simulink library "ESTS_TFY"  (R2023b)
settings: Solver=VariableStepAuto  StartTime=0.0  StopTime=10.0  RelTol=1e-3
libraries: ESTS_TFY_YawMomFromFx x1, ESTS_TFY_LatForceFromFx x1, ESTS_TFY_LatAxle x1, ESTS_TFY_FLatTir x1
settings Model: Creator=blatak  LastModifiedBy=blatak
settings ModelReferenceCC: EnableRefExpFcnMdlSchedulingChecks=on

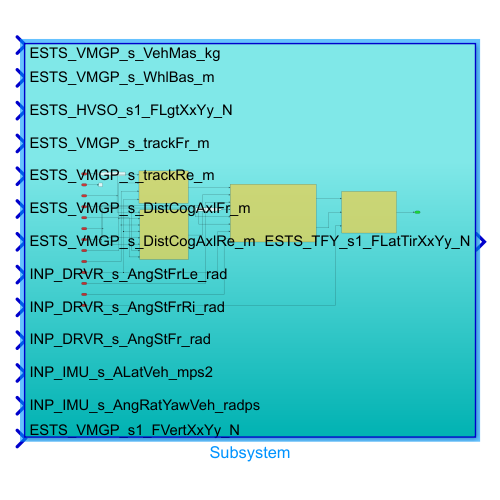
[thumbnail: Simulink's stored preview of the top-level diagram]
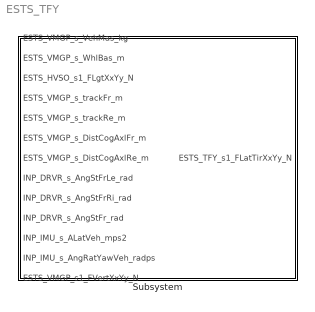
== system ESTS_TFY ==
  Subsystem : Subsystem

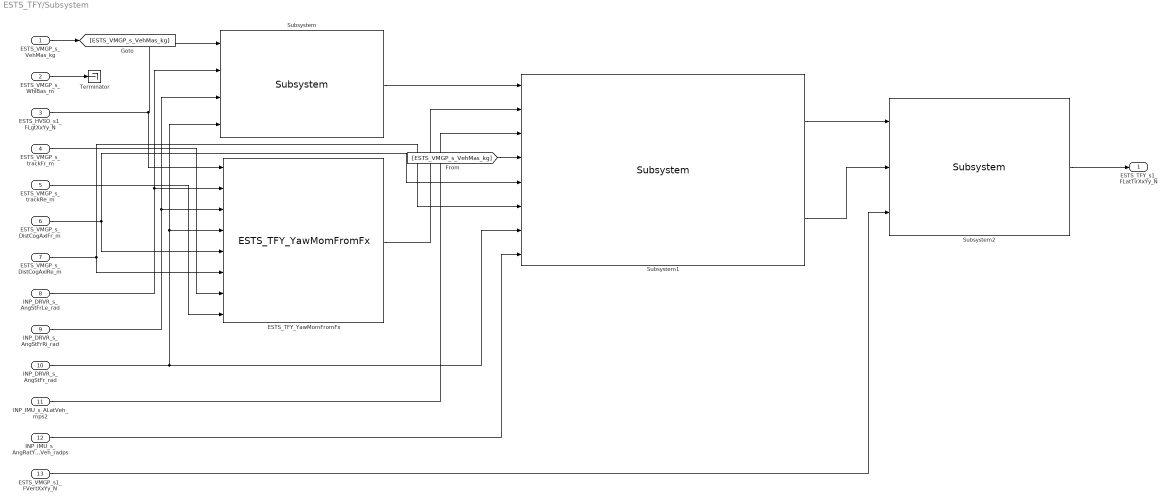
== system ESTS_TFY/Subsystem ==
  ESTS_VMGP_s_VehMas_kg : Inport  Description=Vehicle mass
  ESTS_VMGP_s_WhlBas_m : Inport  Description=Wheelbase - x distance between wheel centers, front to rear  Port=2
  ESTS_HVSO_s1_FLgtXxYy_N : Inport  Description=Estimation of tyre longitudinal forces - vector  Port=3
  ESTS_VMGP_s_trackFr_m : Inport  Description=|  Port=4
      | Front vehicle track - y-distance between tyre contact points left to right, front axle
      | in static position, no change due to kinematic in suspension movement
  ESTS_VMGP_s_trackRe_m : Inport  Description=|  Port=5
      | Rear vehicle track - y-distance between tyre contact points left to right, rear axle
      | in static position, no change due to kinematic in suspension movement
  ESTS_VMGP_s_DistCogAxlFr_m : Inport  Description=X distance from front axle (wheel center) to cog  Port=6
  ESTS_VMGP_s_DistCogAxlRe_m : Inport  Description=X distance from rear axle (wheel center) to cog  Port=7
  INP_DRVR_s_AngStFrLe_rad : Inport  Description=Steering wheel angle FL - calculated only from steering ratio (Ackerman neglected now)  Port=8
  INP_DRVR_s_AngStFrRi_rad : Inport  Description=Steering wheel angle FR - calculated only from steering ratio (Ackerman neglected now)  Port=9
  INP_DRVR_s_AngStFr_rad : Inport  Description=|  Port=10
      | Steering wheel angle front - calculated as an average FL and FR,
      | used for single track model, later more sophisticated calculation method needed 
      | than only an average
  INP_IMU_s_ALatVeh_mps2 : Inport  Description=|  Port=11
      | INP IMU Lateral acceleration - filtered, recalculated to physical value if necessary, 
      | recalculated to cog position, saturated etc.
  INP_IMU_s_AngRatYawVeh_radps : Inport  Description=|  Port=12
      | INP IMU Yaw velocity - filtered, recalculated to physical value if necessary,
      | saturated etc.
  ESTS_VMGP_s1_FVertXxYy_N : Inport  Description=Estimation of vertical wheel loads - vector  Port=13
  ESTS_TFY_YawMomFromFx : ESTS_TFY_YawMomFromFx/ESTS_TFY_YawMomFromFx  SystemSampleTime=-1  VariantActivationTime=update diagram  AllowFlexibleInterface=on  Latency=0  AutoFrameSizeCalculation=off
  Subsystem : ESTS_TFY_LatForceFromFx/Subsystem  SystemSampleTime=-1  VariantActivationTime=update diagram  AllowFlexibleInterface=on  Latency=0  AutoFrameSizeCalculation=off
  Subsystem1 : ESTS_TFY_LatAxle/Subsystem  SystemSampleTime=-1  VariantActivationTime=update diagram  AllowFlexibleInterface=on  Latency=0  AutoFrameSizeCalculation=off
  Subsystem2 : ESTS_TFY_FLatTir/Subsystem  SystemSampleTime=-1  VariantActivationTime=update diagram  AllowFlexibleInterface=on  Latency=0  AutoFrameSizeCalculation=off
  Terminator : Terminator
  ESTS_TFY_s1_FLatTirXxYy_N : Outport  Description=Estimation of tyre lateral forces - vector
  wires:
  Subsystem2/1 -> ESTS_TFY_s1_FLatTirXxYy_N/1
  ESTS_HVSO_s1_FLgtXxYy_N/1 -> ESTS_TFY_YawMomFromFx/1, Subsystem/1
  INP_DRVR_s_AngStFrLe_rad/1 -> ESTS_TFY_YawMomFromFx/2, Subsystem/2
  INP_DRVR_s_AngStFrRi_rad/1 -> ESTS_TFY_YawMomFromFx/3, Subsystem/3
  INP_DRVR_s_AngStFr_rad/1 -> ESTS_TFY_YawMomFromFx/4, Subsystem/4, Subsystem1/7
  ESTS_VMGP_s_DistCogAxlRe_m/1 -> ESTS_TFY_YawMomFromFx/6, Subsystem1/6
  ESTS_VMGP_s_DistCogAxlFr_m/1 -> ESTS_TFY_YawMomFromFx/5, Subsystem1/5
  ESTS_VMGP_s_trackFr_m/1 -> ESTS_TFY_YawMomFromFx/7
  ESTS_VMGP_s_trackRe_m/1 -> ESTS_TFY_YawMomFromFx/8
  Subsystem/1 -> Subsystem1/1
  ESTS_TFY_YawMomFromFx/1 -> Subsystem1/2
  ESTS_VMGP_s_WhlBas_m/1 -> Terminator/1
  INP_IMU_s_ALatVeh_mps2/1 -> Subsystem1/3
  ESTS_VMGP_s_VehMas_kg/1 -> [ESTS_VMGP_s_VehMas_kg]
  [ESTS_VMGP_s_VehMas_kg] -> Subsystem1/4
  INP_IMU_s_AngRatYawVeh_radps/1 -> Subsystem1/8
  Subsystem1/1 -> Subsystem2/1
  Subsystem1/2 -> Subsystem2/2
  ESTS_VMGP_s1_FVertXxYy_N/1 -> Subsystem2/3
